simulink model "equation_mask"  (R2020b)
settings: Solver=VariableStepAuto  StartTime=0.0  StopTime=10.0  RelTol=1e-3
undefined symbols (not defined in the file): c, m
settings Model: Creator=Milind  LastModifiedBy=Milind

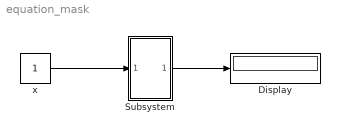
== system equation_mask ==
  Display : Display
  Subsystem : Subsystem
  x : Constant
  wires:
  x/1 -> Subsystem/1(In1)
  Subsystem/1(Out1) -> Display/1

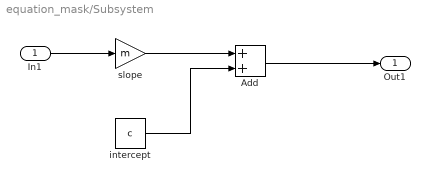
== system equation_mask/Subsystem ==
  In1 : Inport
  Add : Sum
  intercept : Constant  Value=c
  slope : Gain  Gain=m
  Out1 : Outport
  wires:
  slope/1 -> Add/1
  intercept/1 -> Add/2
  Add/1 -> Out1/1
  In1/1 -> slope/1
